simulink model "lab3"  (Simulink 9.1)
settings: Solver=ode45  StartTime=0.0  StopTime=10.0  RelTol=1e-4  EnableMultiTasking=on
values from neighbouring files (symbols this model uses):
  a = 1.55    [Four_1.m]
  b = 10    [Four_1.m]
  K = 32.6    [Four_1.m]
  theta = 0    [Four_1.m]
  TI = 0.0552    [Four_1.m]
  VMAX_UPM = 11.75    [Four_1.m]
settings Model: Creator=maggiore  LastModifiedBy=menonpr7  ExtModeAutoUpdateStatusClock=off
settings DataIOCC: LimitDataPoints=on  SignalLoggingSaveFormat=ModelDataLogs
settings OptimizationCC: ExpressionDepthLimit=2147483647  InitFltsAndDblsToZero=on
settings DebuggingCC: SaveWithParameterizedLinksMsg=none  SignalResolutionControl=TryResolveAllWithWarning  SolverPrmCheckMsg=warning  MultiTaskDSMMsg=warning  MultiTaskCondExecSysMsg=none  FcnCallInpInsideContextMsg=warning  StateNameClashWarn=warning
settings GRTTargetCC: TargetFcnLib=ansi_tfl_tmw.mat  GeneratePreprocessorConditionals=Disable all

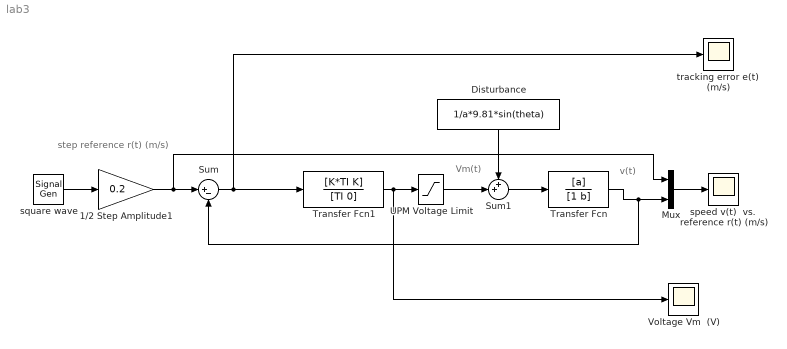
== system lab3 ==
  note: step reference r(t) (m/s)
  note: Vm(t)
  note: v(t)
  1/2 Step Amplitude1 : Gain  Gain=0.2  SaturateOnIntegerOverflow=on  OutDataTypeStr=Inherit: Same as input  ParamDataTypeStr=Inherit: Same as input
  Disturbance : Constant  Value=1/a*9.81*sin(theta)
  Mux : Mux  Inputs=2
  Sum : Sum  Inputs=|+-
  Sum1 : Sum  Inputs=++|
  Transfer Fcn : TransferFcn  Numerator=[a]  Denominator=[1 b]
  Transfer Fcn1 : TransferFcn  Numerator=[K*TI K]  Denominator=[TI 0]
  UPM Voltage Limit : Saturate  UpperLimit=VMAX_UPM  LowerLimit=- VMAX_UPM
  Voltage Vm  (V) : Scope
  speed v(t)  vs.  reference r(t) (m/s) : Scope
  square wave : SignalGenerator  WaveForm=square  Frequency=.5
  tracking error e(t)  (m/s) : Scope
  wires:
  Sum/1 -> tracking error e(t)  (m/s)/1, Transfer Fcn1/1
  square wave/1 -> 1/2 Step Amplitude1/1
  Mux/1 -> speed v(t)  vs.  reference r(t) (m/s)/1
  Transfer Fcn1/1 -> UPM Voltage Limit/1, Voltage Vm  (V)/1
  Sum1/1 -> Transfer Fcn/1
  Disturbance/1 -> Sum1/1
  1/2 Step Amplitude1/1 -> Sum/1, Mux/1
  UPM Voltage Limit/1 -> Sum1/2
  Transfer Fcn/1 -> Mux/2, Sum/2
